simulink model "zynq_dc_motor_control"  (R2019b)
settings: Solver=FixedStepDiscrete  StartTime=0.0  StopTime=inf  RelTol=1e-3  EnableMultiTasking=on
settings Model: SimulationMode=external  Creator=guest  LastModifiedBy=cernylu6
settings DataIOCC: ReturnWorkspaceOutputs=off
settings OptimizationCC: PassReuseOutputArgsAs=Individual arguments  EfficientTunableParamExpr=on
settings DebuggingCC: ParameterTunabilityLossMsg=error  ArithmeticOperatorsInVariantConditions=warning
settings SFSimCC: SimUseLocalCustomCode=off  MATLABDynamicMemAlloc=off  CustomCodeUndefinedFunction=UseInterfaceOnly
settings RTWCC: Description=Linux Embedded Coder  SystemTargetFile=ert_linux.tlc  MakeCommand="make_rtw OPT_OPTS=\"-O2 -ggdb -Wall\" CC=arm-linux-gnueabihf-gcc CPP=arm-linux-gnueabihf-gcc"  TemplateMakefile=ert_linux.tmf  GenerateReport=on  RTWUseLocalCustomCode=off  IncludeHyperlinkInReport=on  LaunchReport=on  GenerateTraceInfo=on  GenerateTraceReport=on  GenerateTraceReportSl=on  GenerateTraceReportSf=on  GenerateTraceReportEml=on
settings CodeAppCC: ForceParamTrailComments=on  IgnoreCustomStorageClasses=off  OperatorAnnotations=on  SimulinkDataObjDesc=on  SFDataObjDesc=on  MATLABFcnDesc=on  InsertBlockDesc=on  StateflowObjectComments=on  MATLABSourceComments=on
settings STFCustomTargetCC: TargetLangStandard=C99 (ISO)  MultiwordLength=256  ModelReferenceCompliant=off  CombineOutputUpdateFcns=on  ERTCustomFileBanners=on  SupportContinuousTime=off  RemoveResetFunc=on  MATLABClassNameForMDSCustomization=Simulink.SoftwareTarget.ERTCustomization  SystemTargetFile=ert_linux.tlc
settings ERTTargetCC: TargetLangStandard=C99 (ISO)  ModelReferenceCompliant=off  ParMdlRefBuildCompliant=off  CompOptLevelCompliant=off  ConcurrentExecutionCompliant=off  SupportNonInlinedSFcns=on  ModelStepFunctionPrototypeControlCompliant=off  CPPClassGenCompliant=off  UseToolchainInfoCompliant=off  ExtMode=on  ExtModeMexArgs='192.168.136.74'  ERTCustomFileTemplate=ert_linux_file_process.tlc

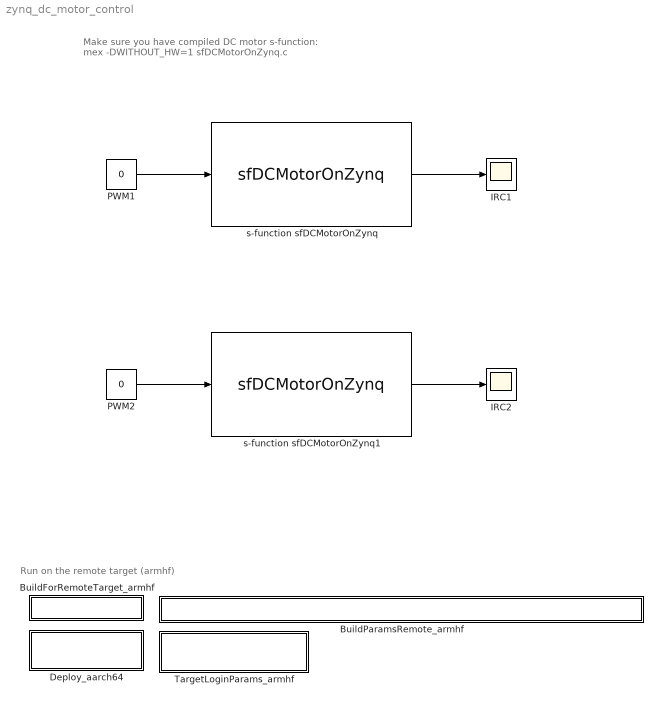
== system zynq_dc_motor_control ==
  note: Make sure you have compiled DC motor s-function:
      | mex -DWITHOUT_HW=1 sfDCMotorOnZynq.c
  note: Run on the remote target (armhf)
  BuildForRemoteTarget_armhf : Subsystem
      settings: OpenFcn=ert_linux_build(gcs, 'BuildParamsRemote_armhf')
      mask Display: disp('Build')
  BuildParamsRemote_armhf : Subsystem  mask{make_command='make_rtw OPT_OPTS="-O2 -ggdb -Wall" CC=arm-linux-gnueabihf-gcc CPP=arm-linux-gnueabihf-gcc'}
      mask prompts: make_command "MakeCommand"
      mask Display: disp(get_param(gcb, 'make_command'));
  Deploy_aarch64 : Subsystem
      settings: OpenFcn=ert_linux_deploy_and_connect(gcs, 'TargetLoginParams_armhf');
      mask Display: disp('Deploy and\nconnect')
  IRC1 : Scope
  IRC2 : Scope
  PWM1 : Constant  Value=0
  PWM2 : Constant  Value=0
  TargetLoginParams_armhf : Subsystem  mask{trgt_ip_addr='192.168.136.74', trgt_username='root'}
      mask prompts: trgt_ip_addr "Target IP address"; trgt_username "Target username"
      mask Display:
      | ip_addr = get_param(gcb, 'trgt_ip_addr');
      | user = get_param(gcb, 'trgt_username');
      | 
      | fprintf('IP addr:\t %s\n User:\t %s ', ip_addr, user);
  s-function sfDCMotorOnZynq : S-Function  FunctionName=sfDCMotorOnZynq  Parameters=Ts,MOT_ID  SFunctionDeploymentMode=off  EnableBusSupport=off  mask{Ts=0.001, MOT_ID=0}
      mask prompts: Ts "Sampling period (Ts):"; MOT_ID "Motor ID:"
      mask help:
      | Input PWM is real number from interval [-1, 1].
      | Output IRC_POS is integer value.
      mask Display:
      | fprintf('MZ_APO DC Motor\ns-function\n(PMOD%d)\n', get_param(gcb, 'MOT_ID')-48);
      | port_label('input', 1, 'PWM')
      | port_label('output',1,'IRC_POS')
  s-function sfDCMotorOnZynq1 : S-Function  FunctionName=sfDCMotorOnZynq  Parameters=Ts,MOT_ID  SFunctionDeploymentMode=off  EnableBusSupport=off  mask{Ts=0.001, MOT_ID=1}
      mask prompts: Ts "Sampling period (Ts):"; MOT_ID "Motor ID:"
      mask help:
      | Input PWM is real number from interval [-1, 1].
      | Output IRC_POS is integer value.
      mask Display:
      | fprintf('MZ_APO DC Motor\ns-function\n(PMOD%d)\n', get_param(gcb, 'MOT_ID')-48);
      | port_label('input', 1, 'PWM')
      | port_label('output',1,'IRC_POS')
  wires:
  PWM1/1 -> s-function sfDCMotorOnZynq/1
  s-function sfDCMotorOnZynq/1 -> IRC1/1
  PWM2/1 -> s-function sfDCMotorOnZynq1/1
  s-function sfDCMotorOnZynq1/1 -> IRC2/1

== system zynq_dc_motor_control/BuildForRemoteTarget_armhf ==

== system zynq_dc_motor_control/BuildParamsRemote_armhf ==

== system zynq_dc_motor_control/Deploy_aarch64 ==

== system zynq_dc_motor_control/TargetLoginParams_armhf ==
